simulink model "checksimobs"  (R2020b)
settings: Solver=FixedStepAuto  StartTime=0.0  StopTime=inf  FixedStep=0.01  RelTol=1e-3
values from neighbouring files (symbols this model uses):
  cc = cc+1    (= 1)    [Path_planning_run.m]    (also in checkpathplaning.m)
  f_stateg = 0    [Path_planning_run.m]    (also in checkpathplaning.m)
  f_statet = 270    [Path_planning_run.m]    (also in checkpathplaning.m = 180)
  f_statex = 60    [Path_planning_run.m]    (also in checkpathplaning.m = 20)
  f_statey = 64    [Path_planning_run.m]    (also in checkpathplaning.m = 40)
  gammad = [-21 0 21]    [Path_planning_run.m]    (also in checkpathplaning.m)
  i_stateg = 0    [Path_planning_run.m]    (also in checkpathplaning.m)
  i_statet = 180    [Path_planning_run.m]    (also in checkpathplaning.m)
  i_statex = 250    [Path_planning_run.m]    (also in checkpathplaning.m = 200)
  i_statey = 45    [Path_planning_run.m]    (also in checkpathplaning.m = 40)
  IC_theta0 = deg2rad(i_statet)+deg2rad(i_stateg)    [Path_planning_run.m]    (also in checkpathplaning.m)
  IC_theta1 = deg2rad(i_statet)    [Path_planning_run.m]    (also in checkpathplaning.m)
  IC_x0 = x_1f-L_0b*cos(IC_theta0)    [Path_planning_run.m]    (also in checkpathplaning.m)
  IC_x1 = i_statex    (= 250)    [Path_planning_run.m]    (also in checkpathplaning.m = 200)
  IC_y0 = y_1f-L_0b*sin(IC_theta0)    [Path_planning_run.m]    (also in checkpathplaning.m)
  IC_y1 = i_statey    (= 45)    [Path_planning_run.m]    (also in checkpathplaning.m = 40)
  idMO = 1    [checkpathplaning.m]
  L_0b = 0.3    [Path_planning_run.m]    (also in boundingbox_AV.m; check3_dyn.m; checkfinal_dyn.m; checkpathplaning.m)
  L_0f = 3.8    [Path_planning_run.m]    (also in boundingbox_AV.m; check3_dyn.m; checkfinal_dyn.m; checkpathplaning.m)
  L_1f = 8.475    [Path_planning_run.m]    (also in boundingbox_AV.m; check3_dyn.m; checkfinal_dyn.m; checkpathplaning.m)
  lookahead_timeforward = 1.5    [Path_planning_run.m]    (also in checkpathplaning.m = 2)
  lookahead_timereverse = 1.5    [Path_planning_run.m]    (also in checkpathplaning.m)
  lv12_0 = hypot((oh_0b),(w_1/2))    [Path_planning_run.m]    (also in boundingbox_AV.m; check3_dyn.m; checkfinal_dyn.m; checkpathplaning.m)
  lv12_1 = hypot(oh_1b,(w_1/2))    [Path_planning_run.m]    (also in boundingbox_AV.m; check3_dyn.m; checkfinal_dyn.m; checkpathplaning.m)
  lv34_0 = hypot((w_1/2),(L_0f+oh_0f))    [Path_planning_run.m]    (also in boundingbox_AV.m; check3_dyn.m; checkfinal_dyn.m; checkpathplaning.m)
  lv34_1 = hypot((w_1/2),oh_1f)    [Path_planning_run.m]    (also in boundingbox_AV.m; check3_dyn.m; checkfinal_dyn.m; checkpathplaning.m)
  MPFpointx = 160    [checkpathplaning.m]    (also in movingobstacledetection.m)
  MPFpointy = MPSpointy+50    (= 75)    [checkpathplaning.m]    (also in movingobstacledetection.m = 85)
  MPSpointx = 160    [checkpathplaning.m]    (also in movingobstacledetection.m)
  MPSpointy = 25    [checkpathplaning.m]    (also in movingobstacledetection.m)
  obsc = 6    [DPDscenario.m]
  oc = 0    [Path_planning_run.m]    (also in checkpathplaning.m)
  oh_0b = 0.94    [Path_planning_run.m]    (also in boundingbox_AV.m; check3_dyn.m; checkfinal_dyn.m; checkpathplaning.m)
  oh_0f = 1.5    [Path_planning_run.m]    (also in boundingbox_AV.m; check3_dyn.m; checkfinal_dyn.m; checkpathplaning.m)
  oh_1b = 5    [Path_planning_run.m]    (also in boundingbox_AV.m; check3_dyn.m; checkfinal_dyn.m; checkpathplaning.m)
  oh_1f = L_1f+1    (= 9.475)    [Path_planning_run.m]    (also in boundingbox_AV.m; check3_dyn.m; checkfinal_dyn.m; checkpathplaning.m)
  steer_ratioforward = 1    [Path_planning_run.m]    (also in checkpathplaning.m)
  steer_ratioreverse = 1    [Path_planning_run.m]    (also in checkpathplaning.m)
  steer_sensforward = 7.7    [Path_planning_run.m]    (also in checkpathplaning.m = 4)
  steer_sensreverse = 7.2    [Path_planning_run.m]    (also in checkpathplaning.m)
  t_MO = deg2rad(90)    [checkpathplaning.m]    (also in movingobstacledetection.m)
  v_0 = 1    [movingobstacledetection.m]
  w_1 = 2.5    [Path_planning_run.m]    (also in boundingbox_AV.m = 10; check3_dyn.m; checkfinal_dyn.m; checkpathplaning.m)
  xv_lc = [x1_lc x2_lc x3_lc x4_lc]    [Path_planning_run.m]    (also in checkpathplaning.m)
  xv_lg = [x1_lg x2_lg x3_lg x4_lg]    [Path_planning_run.m]    (also in checkpathplaning.m; h_costnewslx.m = ppround_1(xv_lg))
  xv_rv = [61.4 30 30 61.4]    [Path_planning_run.m]    (also in checkpathplaning.m)
  yv_lc = [y1_lc y2_lc y3_lc y4_lc]    [Path_planning_run.m]    (also in checkpathplaning.m)
  yv_lg = [y1_lg y2_lg y3_lg y4_lg]    [Path_planning_run.m]    (also in checkpathplaning.m; h_costnewslx.m = ppround_1(yv_lg))
  yv_rv = [20 20 70 70]    [Path_planning_run.m]    (also in checkpathplaning.m)
undefined symbols (not defined in the file or in its folder): DiscIntNeverNeededParam, g, gfin, gini, obsx, obsy, PP_G, PP_T, PP_X, PP_Y, tfin, timeAV, tini, x, xfin, y, yfin
libraries: vrlib x2, simulink x2
(part 3 of 3)

== matlab function checksimobs/Path planner/Path planning algorithm ==
  data: toctime output; cc parameter; f_stateg parameter; g parameter; gammad parameter; gfin parameter; gini parameter; i_stateg parameter; i_statet parameter; i_statex parameter; i_statey parameter; L_0b parameter; L_0f parameter; L_1f parameter; lv12_0 parameter; lv34_0 parameter; obsc parameter; obsx parameter; obsy parameter; oc parameter; oh_0b parameter; oh_0f parameter; oh_1b parameter; oh_1f parameter; t parameter; tfin parameter; timeAV parameter; tini parameter; w_1 parameter; x parameter; xfin parameter; y parameter; yfin parameter; lv12_1 parameter; lv34_1 parameter; path output; xv_lg parameter; yv_lg parameter; f_statex parameter; f_statey parameter; f_statet parameter; xv_rv parameter; yv_rv parameter; xv_lc parameter; yv_lc parameter
function [toctime,path]  = fcn(cc,f_stateg,g, gammad, gfin, gini, i_stateg, i_statet, i_statex, i_statey, L_0b, L_0f, L_1f, lv12_0, lv34_0, obsc, obsx, obsy, oc, oh_0b, oh_0f, oh_1b, oh_1f, t, tfin, timeAV, tini, w_1, x, xfin, y, yfin, lv12_1, lv34_1, xv_lg, yv_lg, f_statex, f_statey, f_statet, xv_rv, yv_rv, xv_lc, yv_lc)
tictime = tic;
%__________________________________________________________________________
coder.extrinsic('Simulink.Bus');
coder.extrinsic('InPolygon');
%__________________________________________________________________________
cur.x = i_statex;
cur.y = i_statey;
cur.xa = i_statex;
cur.ya = i_statey;
cur.pred.tf = i_statet;
cur.pred.gf = i_stateg;
cur.pred.gcost = zeros;
cur.predxy = zeros;
cur.pred.hcost = zeros;
cur.pred.ti = zeros;
cur.pred.gi = zeros;
cur.pred.dir = 1;
%__________________________________________________________________________
ip.x = zeros;
ip.y = zeros;
ip.xa = zeros;
ip.ya = zeros;
ip.pred.ti = zeros;
ip.pred.gi = zeros;
ip.predxy = zeros;
ip.pred.tf  = zeros;
ip.pred.gf  = zeros;
ip.pred.gcost = zeros;
ip.pred.hcost = zeros;
ip.pred.dir = zeros;
%__________________________________________________________________________
t_x     =   zeros(1,200000);     % X config
t_y     =   zeros(1,200000);     % Y config
t_xa    =   zeros(1,200000);     % Actual ending point of MP X
t_ya    =   zeros(1,200000);     % Actual ending point of MP Y
t_predxy    =   zeros(1,200000); % Index of the config before this config in the tree 
t_gcost     =   zeros(1,200000); % Cost so far for this config
t_hcost     =   zeros(1,200000); % Cost to go for this config
t_pred  =   zeros(1,200000);     % Index of the MP used to reach this config
t_dir   =   zeros(1,200000);     % Direction of motion to reach this config
t_count     =   0;  % Count of the explored configs. 
% Adding the initail state in the tree.
t_count     =   t_count+1;
t_x(t_count)=   cur.x;
% asdasd = nonzeros(t_x)
t_y(t_count)=   cur.y;
t_xa(t_count)   =   cur.xa;
t_ya(t_count)   =   cur.ya;
t_predxy(t_count)   =   nan;
t_gcost(t_count)    =   nan;
t_hcost(t_count)    =   nan;
t_pred(t_count) =   nan;
t_dir(t_count)  =   nan;
% open list
o = zeros(1,200000);
oc=oc+1;
o(oc) = t_count;
% closed list
c = zeros(1,200000);
c(cc) = 1;
%__________________________________________________________________________
% % Area definition
% % related to h-cost
% lz_lg = 25;
% wz_lg= 1;
% dt1_lg= f_statet + atand(wz_lg/lz_lg);
% dt2_lg= f_statet - atand(wz_lg/lz_lg);
% dl_lg= hypot(wz_lg/2,lz_lg/2);
% x1_lg=  f_statex + dl_lg*cosd(dt1_lg);
% y1_lg=  f_statey + dl_lg*sind(dt1_lg);
% x2_lg=  f_statex + dl_lg*cosd(dt2_lg);
% y2_lg=  f_statey + dl_lg*sind(dt2_lg);
% x3_lg=  f_statex + dl_lg*cosd(dt1_lg+180);
% y3_lg=  f_statey + dl_lg*sind(dt1_lg+180);
% x4_lg=  f_statex + dl_lg*cosd(dt2_lg+180);
% y4_lg=  f_statey + dl_lg*sind(dt2_lg+180);
% 
% xv_lg = [x1_lg x2_lg x3_lg x4_lg];
% yv_lg = [y1_lg y2_lg y3_lg y4_lg];
% % % % related to h-cost1
% % xv_dv = [61.4 40 40 61.4];
% % yv_dv = [30 30 51 51];
% % related to reversemaneuber
% xv_rv = [61.4 30 30 61.4];
% yv_rv = [20 20 70 70];
% % loopcheck
% lz_lc= 5; % IN zone
% wz_lc= 1.5;
% dt1_lc= f_statet + atand(wz_lc/lz_lc);
% dt2_lc= f_statet - atand(wz_lc/lz_lc);
% dl_lc= hypot(wz_lc/2,lz_lc/2);
% x1_lc=  f_statex + dl_lc*cosd(dt1_lc);
% y1_lc=  f_statey + dl_lc*sind(dt1_lc);
% x2_lc=  f_statex + dl_lc*cosd(dt2_lc);
% y2_lc=  f_statey + dl_lc*sind(dt2_lc);
% x3_lc=  f_statex + dl_lc*cosd(dt1_lc+180);
% y3_lc=  f_statey + dl_lc*sind(dt1_lc+180);
% x4_lc=  f_statex + dl_lc*cosd(dt2_lc+180);
% y4_lc=  f_statey + dl_lc*sind(dt2_lc+180);
% xv_lc = [x1_lc x2_lc x3_lc x4_lc];
% yv_lc = [y1_lc y2_lc y3_lc y4_lc];
%__________________________________________________________________________
loopcheck = 1;
% to have straight path in the upper sector of DPD
xv_rv = [286 30 30 286]; 
yv_rv = [144 144 200 200];

xv_rv1 = [28 0 0 28]; 
yv_rv1 = [60 60 140 140];

xv_rv2 = [286 0 0 286];
yv_rv2 = [0 0 50 50];
while loopcheck 
    condinrv = false(1,1);
    condinrv1 = false(1,1);
    condinrv2 = false(1,1);
    inrv = InPolygon(cur.xa,cur.ya,xv_rv,yv_rv);
    inrv1 = InPolygon(cur.xa,cur.ya,xv_rv1,yv_rv1);
    % % || inrv1==1
%     if inrv==1 || inrv1==1
%         A = [180,270];
%         B = 0;
%     else
        inrv2 = InPolygon(cur.xa,cur.ya,xv_rv2,yv_rv2);
        condinrv = any(inrv);
        condinrv1 = any(inrv1);
        condinrv2 = any(inrv2);
    if condinrv2==1 && i_statey<70 && f_statey>70
        A = [180,90];
        B = 0;
    elseif condinrv==1 && i_statey>70 && f_statey<70
        A = [180,270];
        B = 0;   
    else
        [A1,A2] = virtualforobs_checkslx(cur,obsc,obsx,obsy);
        vthetafor1 = A1;
        vthetafor2 = A2;
        indextoreplace = vthetafor2<0;
        vthetafor2(indextoreplace) = 360+vthetafor2(indextoreplace);
        indextoreplace1 = vthetafor1>=360;
        vthetafor1(indextoreplace1) = vthetafor1(indextoreplace1)-360;
        A6 = [270 342 351 0];
        A = horzcat(vthetafor1,vthetafor2,A6);
%     A = horzcat(vthetafor1,vthetafor2);
        B = gammad;
    end
    checkti     = cur.pred.tf==tini;
    checkgi     = cur.pred.gf==gini;
    checktif    = ismember(tfin,A);
    checkgif    = ismember(gfin,B);
    cond        =   all([checkti;checkgi;checktif;checkgif]); 
    index       =   find(cond);
    ifcheck     =   ~isempty(index);
    if ifcheck
        for k   =   1:length(index) 
            ip.pred.ti  =   cur.pred.tf;
            ip.pred.gi  =   cur.pred.gf;
            % replacing c(cc) by other variable - check
%             check10 = c(cc);
%             check10_1 = nonzeros(check10)
            ip.predxy   =   c(cc);
%             ip.predxy   =   check10_1;
            if cur.pred.dir     ==  1 
                ip.pred.dir=1;
            end
            if cur.pred.dir     ==  0
                ip.pred.dir=1;
            end 
            xp   = x(:,index(k));
            yp   = y(:,index(k));
            thetap = t(:,index(k));
            gammap = g(:,index(k));
            dirp   = ip.pred.dir;
            ip.xa = cur.xa+xp(length(xp)); 
            ip.ya = cur.ya+yp(length(yp));
            ip.pred.tf  =   tfin(index(k));
            ip.pred.gf  =   gfin(index(k));
            pathlength = timeAV(index(k));
            ip.x = ppround_1(ip.xa);
            ip.y = ppround_1(ip.ya);
            check_c       = closed_checkCopy(t_x,t_y,c,ip);
            check_obstacle = staticobs_checkCopy(cur,xp,yp,thetap,gammap,dirp,obsc,obsx,obsy,L_0b,L_0f,L_1f,lv12_0,lv34_0,oh_0b,oh_0f,oh_1b,oh_1f,w_1,lv12_1,lv34_1);
            if check_c && check_obstacle
                ip.pred.gcost = g_costCopy(cur,pathlength);
                ip.pred.hcost = h_costnewslx(ip,xv_lg,yv_lg,f_statet,f_statex,f_statey,i_statey);
                check_o       = open_checkCopy(t_x,t_y,t_gcost,ip,o,oc);
                if check_o
                    % Adding the state to the tree
                    t_count=t_count+1;
                    t_x(t_count)= ip.x;
                    t_y(t_count)= ip.y;
                    t_predxy(t_count)= ip.predxy;
                    t_xa(t_count)= ip.xa;
                    t_ya(t_count)= ip.ya;
                    t_pred(t_count)= index(k);
                    t_dir(t_count)= ip.pred.dir;
                    t_gcost(t_count)= ip.pred.gcost;
                    t_hcost(t_count)= ip.pred.hcost;
                    oc=oc+1;                                                % Updating open count
                    o(oc)=t_count;
                end
            end
        end
    end
   %_______________________________________________________________________
   % Reverse path
%    condrev = false(1,1);    % initialise as logical array
%    inrv = InPolygon(cur.xa,cur.ya,xv_rv,yv_rv);
%    condrev = any(inrv);
%     if condrev==1
%         checkti= cur.pred.tf==tfin;                                             % Selecting MP with initial states equal to the final state of the previous config but with tfin and gfin (reverse)
%         checkgi= cur.pred.gf==gfin;
%         cond = all([checkti;checkgi]);                                        % Finding indexes of those MP in the MP bank
%         index= find(cond);
%     else
%         checkti= cur.pred.tf==tfin;                                             % Selecting MP with initial states equal to the final state of the previous config but with tfin and gfin (reverse)
%         checkgi= cur.pred.gf==gfin;
%         checktif= cur.pred.tf==tini;                                          % This is done because the matrix dimensions didn't match if we use previous logical condition
%         checkgif= cur.pred.gf==gini;                                        % This is done because the matrix dimensions didn't match if we use previous logical condition
%         cond = all([checkti;checkgi;checktif;checkgif]);                 % Finding indexes of those MP in the MP bank
%         index= find(cond); 
%     end
   [A3,A4] = virtualobsreverse_checkCopy(cur,obsc,obsx,obsy,oh_1b,oh_1f,w_1,lv12_1,lv34_1);
   vthetarev1 = A3;
   vthetarev2 = A4;
   indextoreplace = vthetarev2<0; 
   vthetarev2(indextoreplace) = 360+vthetarev2(indextoreplace);
   indextoreplace1 = vthetarev1>=360;
   vthetarev1(indextoreplace1) = vthetarev1(indextoreplace1)-360;
   A5 = [270 90];
   AR = horzcat(vthetarev1,vthetarev2,A5);
   B = gammad;    
   checkti= cur.pred.tf==tfin;  
   checkgi= cur.pred.gf==gfin;
   checktif    = ismember(tini,AR); 
   checkgif    = ismember(gini,B);     
   cond        = all([checkti;checkgi;checktif;checkgif]);
   index= find(cond);    
   ifcheck = ~isempty(index);
   if ifcheck
       for k=1:length(index)
           ip.pred.ti  =   cur.pred.tf;
           ip.pred.gi  =   cur.pred.gf;
           % replacing c(cc) by other variable - check
%             check10 = c(cc);
%             check10_1 = nonzeros(check10);
            ip.predxy   =   c(cc);
%             ip.predxy   =   check10_1;
           if cur.pred.dir==1
               ip.pred.dir=0;
           end
           if cur.pred.dir==0
               ip.pred.dir=0;
           end
           xp=x(:,index(k));
           yp=y(:,index(k));
           xfinr=xfin(index(k));
           yfinr=yfin(index(k));
           xp=xp-xfinr;
           yp=yp-yfinr; 
           thetap = t(:,index(k));
           gammap = g(:,index(k));
           dirp   = ip.pred.dir;
           pathlength = timeAV(index(k));
           ip.xa = cur.xa+xp(1);  
           ip.ya = cur.ya+yp(1); 
           ip.pred.tf  =   tini(index(k));
           ip.pred.gf  =   gini(index(k));
           ip.x = ppround_1(ip.xa);
           ip.y = ppround_1(ip.ya);
           check_c       = closed_checkCopy(t_x,t_y,c,ip); 
           check_obstacle = staticobs_checkCopy(cur,xp,yp,thetap,gammap,dirp,obsc,obsx,obsy,L_0b,L_0f,L_1f,lv12_0,lv34_0,oh_0b,oh_0f,oh_1b,oh_1f,w_1,lv12_1,lv34_1);
           if check_c && check_obstacle
               ip.pred.gcost = g_costCopy(cur,pathlength);
               ip.pred.hcost = h_costnewslx(ip,xv_lg,yv_lg,f_statet,f_statex,f_statey,i_statey);
               check_o       = open_checkCopy(t_x,t_y,t_gcost,ip,o,oc);
               if check_o
                   t_count=t_count+1;
                    t_x(t_count)= ip.x;
                    t_y(t_count)= ip.y;
                    t_predxy(t_count)= ip.predxy;
                    t_xa(t_count)= ip.xa;
                    t_ya(t_count)= ip.ya;
                    t_pred(t_count)= index(k);
                    t_dir(t_count)= ip.pred.dir;
                    t_gcost(t_count)= ip.pred.gcost;
                    t_hcost(t_count)= ip.pred.hcost;
                    oc=oc+1;
                    o(oc)=t_count;
               end
           end
       end
   end
   ocopy1 = nonzeros(o);
   ocopy2 = ocopy1';
%    ocopy3 = rmmissing(ocopy2);
   tcostall= t_gcost(ocopy2)+t_hcost(ocopy2);
   [~,min_ind]    = min(tcostall);
   cc         =   cc+1;
%    % check this once
   c(cc)      =   ocopy2(min_ind);
   j=o==(c(cc));
    o(j)=zeros(1,1);
%    o(min_ind) =   zeros;
%    o = rmmissing(o);
% %    o = sds;
%    oc         =   oc-1;
% %    %_______________________________________________________________________
%    % Plot the explored graph real-time (to be deleted)
%    index        =   t_pred(c(cc));
%     if t_dir(c(cc))==1
%         xp=x(:,index);
%         yp   = y(:,index);
%     else
%         xp=x(:,index)-xfin(index);
%         yp=y(:,index)-yfin(index);
%     end
%     thetap = t(:,index);
%     gammap = g(:,index);
%     dirp   = t_dir(c(cc));
%     pred_index= t_predxy(c(cc));
%     xp= xp+t_xa(pred_index);
%     yp= yp+t_ya(pred_index);
%     plot(xp,yp);
%     drawnow
%     hold on;
% %     
    cur.x           =   t_x(c(cc));                                         % Initializing cur to minimum cost state
    cur.y           =   t_y(c(cc));
    cur.xa          =   t_xa(c(cc));
    cur.ya          =   t_ya(c(cc));
    cur.predxy      =   t_predxy(c(cc));
    index           =   t_pred(c(cc));
    cur.pred.dir    =   t_dir(c(cc)); 
    cur.pred.hcost  =   t_hcost(c(cc));
    cur.pred.gcost  =   t_gcost(c(cc));
    if cur.pred.dir == 1
        cur.pred.ti     =   tini(index);
        cur.pred.gi     =   gini(index);
        cur.pred.tf     =   tfin(index);
        cur.pred.gf     =   gfin(index);
    else
        cur.pred.ti     =   tfin(index);
        cur.pred.gi     =   gfin(index);
        cur.pred.tf     =   tini(index);
        cur.pred.gf     =   gini(index);   
    end
%    
    loopcheck   = loop_checkfinalslx(cur,xv_lc,yv_lc,f_statet,f_stateg);
end

%__________________________________________________________________________

% 'L0b'  = +ve, indicates that the respective kingpin is ahead of tractor
% drive axle (Fifth-wheel coupling)
% 'L0b'  = -ve, indicates that the respective kingpin is behind the tractor
% drive axle (Draw-bar coupling)

%__________________________________________________________________________

% Extracting the reference path from the path planner
indexp  =   c(cc);
indexmp =   t_pred(indexp);
% Creating arrays to store path information
pathx = zeros(21,20);
pathy = zeros(21,20);
i = 0;
pathdir = zeros(1,20);
% pathtfin = zeros(21,20);
paththeta = zeros(21,20);
pathgamma = zeros(21,20);
% Extracting a path information from the tree
while (t_x(indexp)~= i_statex || t_y(indexp) ~= i_statey)&& ~isnan(indexmp)
    xp  =   x(:,indexmp);
    yp  =   y(:,indexmp);
    thetap = t(:,indexmp);
    gammap = g(:,indexmp);
%     thetap  =   tfin(indexmp);
    dirp    =   t_dir(indexp);
    pred_index  =   t_predxy(indexp);
    if dirp==1
        xp= xp+t_xa(pred_index);
        yp= yp+t_ya(pred_index);
        figure(1);
        plot(xp,yp,'r');
        drawnow
    else
        xp=xp-xp(length(xp))+t_xa(pred_index);
        yp=yp-yp(length(yp))+t_ya(pred_index);
        xp=flip(xp);
        yp=flip(yp);  
        
        figure(1);
        plot(xp,yp,'-r');
        drawnow
    end
    figure(1);
    plot(xp,yp,'r','linewidth',1.5);
    drawnow
    i   =   i+1;            % Array index
    pathx(:,i)  =   xp;    % Storing path information                                                             
    pathy(:,i)  =   yp;
    pathdir(i)  =   dirp;
    paththeta(:,i) = thetap;
    pathgamma(:,i) = gammap;
%     pathtfin(i) =   thetap;
    indexp      =   t_predxy(indexp);
    indexmp     =   t_pred(indexp);
end
% pathdircheck = nonzeros(pathdir);   % remove zeros from the path direction array
% pathdircheck1 = pathdircheck';      
path = nan(1000,5);
k = 1;
for m = i:-1:1
    for j = 1:21
        path(k,1) = pathx(j,m);
        path(k,2) = pathy(j,m);
        path(k,3) = pathdir(:,m);
        path(k,4) = paththeta(j,m);
        path(k,5) = pathgamma(j,m);
        k = k+1;
    end
end

toctime=toc(tictime);
